simulink model "SendFetchS2"  (Simulink 7.1)
settings: Solver=FixedStepDiscrete  StartTime=0.0  StopTime=inf  FixedStep=0.1  RelTol=1e-3
(part 1 of 2)
settings Model: Creator=kthwsnt  LastModifiedBy=kthwsnt

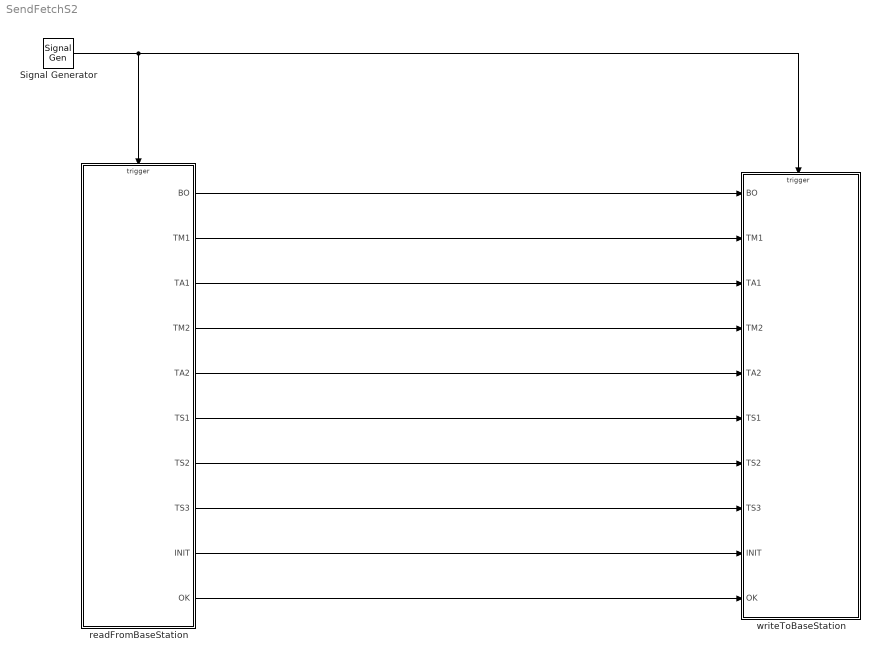
== system SendFetchS2 ==
  Signal Generator : SignalGenerator  WaveForm=square
  readFromBaseStation : Subsystem  TreatAsAtomicUnit=on
  writeToBaseStation : Subsystem  TreatAsAtomicUnit=on
  wires:
  Signal Generator/1 -> readFromBaseStation/Trigger, writeToBaseStation/Trigger
  readFromBaseStation/1(BO) -> writeToBaseStation/1(BO)
  readFromBaseStation/2(TM1) -> writeToBaseStation/2(TM1)
  readFromBaseStation/3(TA1) -> writeToBaseStation/3(TA1)
  readFromBaseStation/4(TM2) -> writeToBaseStation/4(TM2)
  readFromBaseStation/5(TA2) -> writeToBaseStation/5(TA2)
  readFromBaseStation/6(TS1) -> writeToBaseStation/6(TS1)
  readFromBaseStation/7(TS2) -> writeToBaseStation/7(TS2)
  readFromBaseStation/8(TS3) -> writeToBaseStation/8(TS3)
  readFromBaseStation/9(INIT) -> writeToBaseStation/9(INIT)
  readFromBaseStation/10(OK) -> writeToBaseStation/10(OK)

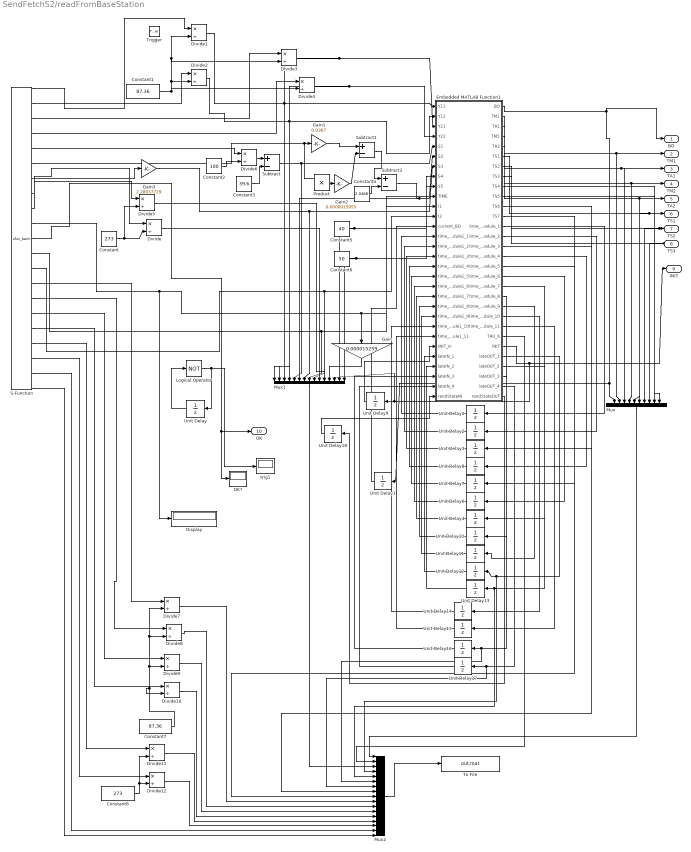
== system SendFetchS2/readFromBaseStation ==
  Trigger : TriggerPort
  Constant : Constant  Value=273  OutDataType=sfix(16)  OutScaling=2^0
  Constant1 : Constant  Value=87.36  OutDataType=sfix(16)  OutScaling=2^0
  Constant2 : Constant  Value=100  OutDataType=sfix(16)  OutScaling=2^0
  Constant3 : Constant  Value=39.6  OutDataType=sfix(16)  OutScaling=2^0
  Constant4 : Constant  Value=2.0468  OutDataType=sfix(16)  OutScaling=2^0
  Constant5 : Constant  Value=40  OutDataType=sfix(16)  OutScaling=2^0
  Constant6 : Constant  Value=50  OutDataType=sfix(16)  OutScaling=2^0
  Constant7 : Constant  Value=87.36  OutDataType=sfix(16)  OutScaling=2^0
  Constant8 : Constant  Value=273  OutDataType=sfix(16)  OutScaling=2^0
  Display : Display
  Divide{,1..12} (13 alike) : Product  Inputs=*/  OutDataType=sfix(16)  OutScaling=2^-10
  Embedded MATLAB Function1 : Stateflow chart
  Gain : Gain  Orientation=down  Gain=0.000015259  ParameterDataType=sfix(16)  ParameterScaling=2^0  OutDataType=sfix(16)  OutScaling=2^0
  Gain1 : Gain  Gain=0.0367  ParameterDataType=sfix(16)  ParameterScaling=2^0  OutDataType=sfix(16)  OutScaling=2^0
  Gain2 : Gain  Gain=0.0000015955  ParameterDataType=sfix(16)  ParameterScaling=2^0  OutDataType=sfix(16)  OutScaling=2^0
  Gain3 : Gain  Gain=2.28937729  ParameterDataType=sfix(16)  ParameterScaling=2^0  OutDataType=sfix(16)  OutScaling=2^0
  Logical Operator : Logic  Operator=NOT  AllPortsSameDT=off  OutDataTypeMode=boolean  OutDataTypeStr=boolean
  Mux : Mux  Orientation=down  Inputs=10
  Mux1 : Mux  Orientation=down  Inputs=15
  Mux2 : Mux  Inputs=17
  OK? : Display
  Product : Product  OutDataType=sfix(16)  OutScaling=2^0  RndMeth=Zero
  S-Function : S-Function  FunctionName=sfun_fetch  SFunctionModules='sfsource'  EnableBusSupport=off
  Subtract : Sum  Inputs=+-  OutDataType=sfix(16)  OutScaling=2^-10
  Subtract1 : Sum  Inputs=+-  OutDataType=sfix(16)  OutScaling=2^-10
  Subtract2 : Sum  Inputs=+-  OutDataType=sfix(16)  OutScaling=2^-10
  To File : ToFile  Filename=out.mat  MatrixName=data
  Unit Delay{,2..17} (17 alike) : UnitDelay  Orientation=left  SampleTime=-1
  Unit Delay1 : UnitDelay  Orientation=left  X0=6  SampleTime=-1
  Unit Delay18 : UnitDelay  Orientation=left  X0=5478.07  SampleTime=-1
  trig1 : Display
  BO : Outport  OutDataType=sfix(16)  OutScaling=2^0
  TM1 : Outport  Port=2  OutDataType=sfix(16)  OutScaling=2^0
  TA1 : Outport  Port=3  OutDataType=sfix(16)  OutScaling=2^0
  TM2 : Outport  Port=4  OutDataType=sfix(16)  OutScaling=2^0
  TA2 : Outport  Port=5  OutDataType=sfix(16)  OutScaling=2^0
  TS1 : Outport  Port=6  OutDataType=sfix(16)  OutScaling=2^0
  TS2 : Outport  Port=7  OutDataType=sfix(16)  OutScaling=2^0
  TS3 : Outport  Port=8  OutDataType=sfix(16)  OutScaling=2^0
  INIT : Outport  Port=9  OutDataType=sfix(16)  OutScaling=2^0
  OK : Outport  Port=10  OutDataType=sfix(16)  OutScaling=2^0
  wires:
  S-Function/11 -> OK?/1, OK/1
  Constant/1 -> Divide/2, Divide5/2
  Divide/1 -> Mux1/10
  S-Function/8 -> Divide/1
  Constant1/1 -> Divide2/2, Divide1/2, Divide3/2, Divide4/2
  S-Function/1 -> Divide1/1
  Divide1/1 -> Embedded MATLAB Function1/1(Y11), Mux1/1
  S-Function/2 -> Divide2/1
  Divide2/1 -> Embedded MATLAB Function1/2(Y12), Mux1/2
  S-Function/12 -> Embedded MATLAB Function1/11(I1), Mux1/8
  S-Function/13 -> Embedded MATLAB Function1/12(I2), Mux1/9
  S-Function/10 -> Display/1, Embedded MATLAB Function1/10(TIME), Gain/1
  Logical Operator/1 -> Unit Delay/1, trig1/1
  Unit Delay/1 -> Logical Operator/1
  Unit Delay1/1 -> Embedded MATLAB Function1/13(current_BO)
  Mux/1 -> Mux2/1
  Mux2/1 -> To File/1
  Embedded MATLAB Function1/1(BO) -> BO/1, Mux/1, Unit Delay1/1
  Embedded MATLAB Function1/2(TM1) -> TM1/1, Mux/2
  Embedded MATLAB Function1/3(TA1) -> TA1/1, Mux/3
  Embedded MATLAB Function1/4(TM2) -> TM2/1, Mux/4
  Embedded MATLAB Function1/5(TA2) -> TA2/1, Mux/5
  Embedded MATLAB Function1/6(TS1) -> TS1/1, Mux/6
  Embedded MATLAB Function1/7(TS2) -> TS2/1, Mux/7
  Embedded MATLAB Function1/8(TS3) -> TS3/1, Mux/8
  Embedded MATLAB Function1/13(time_schedule_1) -> Unit Delay5/1
  Embedded MATLAB Function1/14(time_schedule_2) -> Unit Delay2/1
  Embedded MATLAB Function1/15(time_schedule_3) -> Unit Delay3/1
  Embedded MATLAB Function1/16(time_schedule_4) -> Unit Delay8/1
  Embedded MATLAB Function1/17(time_schedule_5) -> Unit Delay7/1
  Embedded MATLAB Function1/18(time_schedule_6) -> Unit Delay6/1
  Embedded MATLAB Function1/19(time_schedule_7) -> Unit Delay4/1
  Unit Delay5/1 -> Embedded MATLAB Function1/14(time_schedule1_1)
  Unit Delay2/1 -> Embedded MATLAB Function1/15(time_schedule1_2)
  Unit Delay3/1 -> Embedded MATLAB Function1/16(time_schedule1_3)
  Unit Delay8/1 -> Embedded MATLAB Function1/17(time_schedule1_4)
  Unit Delay7/1 -> Embedded MATLAB Function1/18(time_schedule1_5)
  Unit Delay6/1 -> Embedded MATLAB Function1/19(time_schedule1_6)
  Unit Delay4/1 -> Embedded MATLAB Function1/20(time_schedule1_7)
  Gain/1 -> Mux1/12
  S-Function/3 -> Divide3/1
  Divide3/1 -> Embedded MATLAB Function1/3(Y21), Mux1/3
  S-Function/4 -> Divide4/1
  Divide4/1 -> Embedded MATLAB Function1/4(Y22), Mux1/4
  S-Function/9 -> Divide5/1
  Divide5/1 -> Mux1/11
  Constant2/1 -> Divide6/2
  S-Function/5 -> Divide6/1
  Divide6/1 -> Subtract/1
  Constant3/1 -> Subtract/2
  Subtract/1 -> Embedded MATLAB Function1/5(S1), Mux1/5
  S-Function/6 -> Gain1/1, Product/1, Product/2
  Product/1 -> Gain2/1
  Gain1/1 -> Subtract1/1
  Gain2/1 -> Subtract1/2
  Constant4/1 -> Subtract2/2
  Subtract1/1 -> Subtract2/1
  Subtract2/1 -> Embedded MATLAB Function1/6(S2), Mux1/6
  S-Function/7 -> Gain3/1
  Gain3/1 -> Embedded MATLAB Function1/7(S3), Mux1/7
  Mux1/1 -> Mux2/3
  Embedded MATLAB Function1/25(INIT) -> INIT/1, Unit Delay9/1, Mux1/13
  Unit Delay9/1 -> Embedded MATLAB Function1/25(INIT_in)
  Embedded MATLAB Function1/9(TS4) -> Mux/9
  Embedded MATLAB Function1/10(TS5) -> Mux/10
  Constant5/1 -> Embedded MATLAB Function1/8(S4), Mux1/14
  Constant6/1 -> Embedded MATLAB Function1/9(S5), Mux1/15
  Embedded MATLAB Function1/20(time_schedule_8) -> Unit Delay10/1
  Embedded MATLAB Function1/21(time_schedule_9) -> Unit Delay11/1
  Embedded MATLAB Function1/26(lateOUT_1) -> Unit Delay12/1, Mux2/4
  Embedded MATLAB Function1/27(lateOUT_2) -> Unit Delay13/1, Mux2/5
  Unit Delay10/1 -> Embedded MATLAB Function1/21(time_schedule1_8)
  Unit Delay11/1 -> Embedded MATLAB Function1/22(time_schedule1_9)
  Unit Delay12/1 -> Embedded MATLAB Function1/26(lateIN_1)
  Unit Delay13/1 -> Embedded MATLAB Function1/27(lateIN_2)
  Embedded MATLAB Function1/24(TAU_K) -> Mux2/2
  Embedded MATLAB Function1/22(time_schedule_10) -> Unit Delay14/1
  Embedded MATLAB Function1/23(time_schedule_11) -> Unit Delay15/1
  Embedded MATLAB Function1/28(lateOUT_3) -> Unit Delay16/1, Mux2/6
  Embedded MATLAB Function1/29(lateOUT_4) -> Unit Delay17/1, Mux2/7
  Unit Delay14/1 -> Embedded MATLAB Function1/23(time_schedule1_10)
  Unit Delay15/1 -> Embedded MATLAB Function1/24(time_schedule1_11)
  Unit Delay16/1 -> Embedded MATLAB Function1/28(lateIN_3)
  Unit Delay17/1 -> Embedded MATLAB Function1/29(lateIN_4)
  Embedded MATLAB Function1/11(TS6) -> Mux2/8
  Embedded MATLAB Function1/12(TS7) -> Mux2/9
  Unit Delay18/1 -> Embedded MATLAB Function1/30(randStateIN)
  Embedded MATLAB Function1/30(randStateOUT) -> Unit Delay18/1
  S-Function/14 -> Divide7/1
  S-Function/15 -> Divide8/1
  S-Function/16 -> Divide9/1
  S-Function/17 -> Divide10/1
  S-Function/18 -> Divide11/1
  S-Function/19 -> Divide12/1
  S-Function/20 -> Mux2/16
  S-Function/21 -> Mux2/17
  Constant7/1 -> Divide7/2, Divide8/2, Divide9/2, Divide10/2
  Divide7/1 -> Mux2/10
  Divide8/1 -> Mux2/11
  Divide9/1 -> Mux2/12
  Divide10/1 -> Mux2/13
  Constant8/1 -> Divide12/2, Divide11/2
  Divide11/1 -> Mux2/14
  Divide12/1 -> Mux2/15

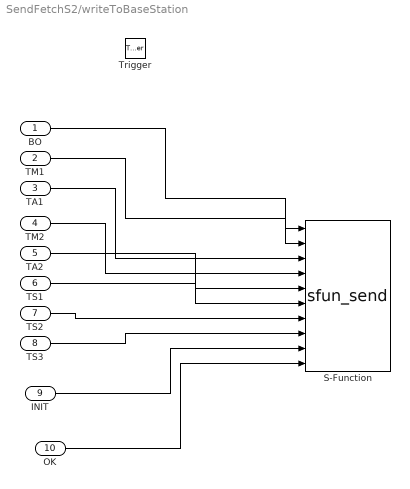
== system SendFetchS2/writeToBaseStation ==
  BO : Inport  OutDataType=sfix(16)  OutScaling=2^0
  TM1 : Inport  Port=2  OutDataType=sfix(16)  OutScaling=2^0
  TA1 : Inport  Port=3  OutDataType=sfix(16)  OutScaling=2^0
  TM2 : Inport  Port=4  OutDataType=sfix(16)  OutScaling=2^0
  TA2 : Inport  Port=5  OutDataType=sfix(16)  OutScaling=2^0
  TS1 : Inport  Port=6  OutDataType=sfix(16)  OutScaling=2^0
  TS2 : Inport  Port=7  OutDataType=sfix(16)  OutScaling=2^0
  TS3 : Inport  Port=8  OutDataType=sfix(16)  OutScaling=2^0
  INIT : Inport  Port=9  OutDataType=sfix(16)  OutScaling=2^0
  OK : Inport  Port=10  OutDataType=sfix(16)  OutScaling=2^0
  Trigger : TriggerPort  TriggerType=falling
  S-Function : S-Function  FunctionName=sfun_send  SFunctionModules='sfsource'  EnableBusSupport=off
  wires:
  BO/1 -> S-Function/1
  TM1/1 -> S-Function/2
  TA1/1 -> S-Function/3
  TM2/1 -> S-Function/4
  TA2/1 -> S-Function/5
  TS1/1 -> S-Function/6
  TS2/1 -> S-Function/7
  TS3/1 -> S-Function/8
  INIT/1 -> S-Function/9
  OK/1 -> S-Function/10
